simulink model "version13"  (Simulink 8.3)
settings: Solver=ode4  StartTime=0  StopTime=60  FixedStep=0.001  MaxStep=0.01  MinStep=0.005  RelTol=1e-3
values from neighbouring files (symbols this model uses):
  Actuator_Tg = 0.1    [init.m]
  airDensity = [1.225 1.0066 .81935 .66011 .52579 .41351 .31194 .22786 .16647 .12165 .08891 .040084 .01841 .0084634 .0039957 .0019663 .0010269 .0005681 .00030968 .00016321 .000082829 .000039921 .000018458 .0000082196 .000003416 .0000005604 .00000009708 .00000002222 .000000008152 .000000003831 .000000002076 .000000001233 .0000000007815 .0000000005194 .0000000003581 .0000000002541 .0000000001367 .00000000007858 .0 ...(+113 chars)    [init.m]
  alphaRange = [-30, -25, -20, -15, -12, -10, -8, -6, -4, -2, 0, 2, 4, 6, 8, 10, 12, 15, 20, 25, 30]    [init.m]
  betaRange = alphaRange    [init.m]
  Cmy_beta = Cmz_alpha    [init.m]
  Cz = Cy    [init.m]
  D = 0.122    [init.m]
  deltayRange = deltazRange    [init.m]
  deltazRange = [-20, -15, -10, -5, 0, 5, 10, 15, 20]    [init.m]
  fai0 = 0    [init.m]
  fai_v0 = 0    [init.m]
  g = 9.8    [init.m]
  gama0 = 0    [init.m]
  h = [0 2 4 6 8 10 12 14 16 18 20 25 30 35 40 45 50 55 60 65 70 75 80 85 90 100 110 120 130 140 150 160 170 180 190 200 220 240 260 280 300 400 500 600 700 800 900]    [init.m]
  Ixx = linspace(0.007,0.006,length(P))    [init.m]
  Iyy = linspace(1.0920,0.7440,length(P))    [init.m]
  K = 4    [init.m]
  Kd_ny = 5    [init.m]
  Kp_gamma = 5    [init.m]
  Kp_ny = 5    [init.m]
  Kp_nz = 5    [init.m]
  L = 1.2    [init.m]
  m = linspace(12+2,9.2,length(P))    [init.m]
  MachRange = [0.6, 1.2, 1.5, 1.8, 2.2]    [init.m]
  Mx_wx = zeros(1,11)    [init.m]
  My_wy = zeros(1,11)    [init.m]
  Mz_wz = zeros(1,11)    [init.m]
  P = 0:0.5:t_propshutdown    [init.m]
  sit0 = angle/57.3    (= 0.139616055846)    [init.m]
  Sref = 0.0038465    [init.m]
  t_change = 0:0.5:t_propshutdown    [init.m]
  t_masschange = 9.5    [init.m]
  t_propshutdown = 9.5    [init.m]
  Tg = 0.5    [init.m]
  theta0 = angle/57.3    (= 0.139616055846)    [init.m]
  V0 = 0.6*340    (= 204)    [init.m]
  Vt = 200    [init.m]
  wx0 = 0    [init.m]
  wy0 = 0    [init.m]
  wz0 = 0    [init.m]
  x0 = 0    [init.m]
  xt0 = 2500    [init.m]
  y0 = 5000    [init.m]
  yt0 = 5000    [init.m]
  z0 = 0    [init.m]
  zt0 = 0    [init.m]
undefined symbols (not defined in the file or in its folder): Cmz_alpha, Cx, Cy, earthRadius
settings Model: Creator=Administrator  LastModifiedBy=answer
settings SolverCC: InitialStep=0.005
settings OptimizationCC: ExpressionDepthLimit=2147483647  InitFltsAndDblsToZero=on
settings DebuggingCC: AlgebraicLoopMsg=none  SaveWithParameterizedLinksMsg=none  SignalResolutionControl=TryResolveAllWithWarning  MultiTaskDSMMsg=warning  MultiTaskCondExecSysMsg=none  FcnCallInpInsideContextMsg=UseLocalSettings
settings SFSimCC: SimParseCustomCode=off
settings RTWCC: IncludeERTFirstTime=on
settings GRTTargetCC: TargetFcnLib=ansi_tfl_tmw.mat

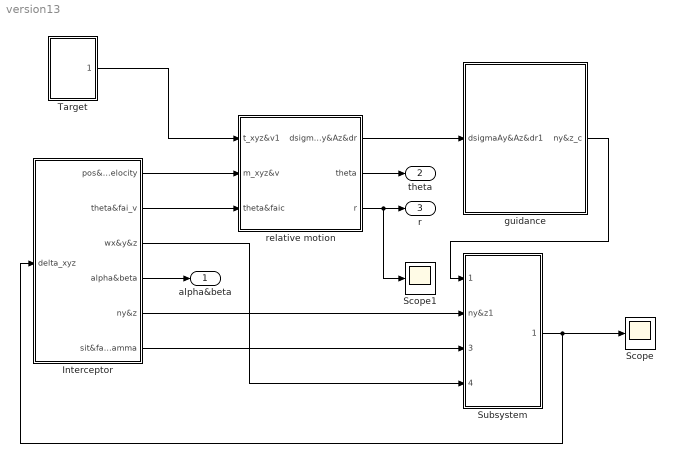
== system version13 ==
  Interceptor : Subsystem
  Scope : Scope
      settings: TimeRange=240  SaveName=ScopeData34
  Scope1 : Scope
      settings: TimeRange=240  SaveName=ScopeData41
  Subsystem : Subsystem
  Target : Subsystem
  guidance : Subsystem
  "relative motion " : Subsystem
  alpha&beta : Outport
  theta : Outport  Port=2
  r : Outport  Port=3
  wires:
  Subsystem/1("delta_xyz1 ") -> Interceptor/1(delta_xyz), Scope/1
  Interceptor/1(pos&velocity) -> "relative motion "/2(m_xyz&v)
  Interceptor/2(theta&fai_v) -> "relative motion "/3(theta&faic)
  Interceptor/4(alpha&beta) -> alpha&beta/1
  Target/1(t_xyz&v) -> "relative motion "/1(t_xyz&v1)
  "relative motion "/2(theta) -> theta/1
  "relative motion "/3(r) -> Scope1/1, r/1
  "relative motion "/1(dsigmaAy&Az&dr) -> guidance/1(dsigmaAy&Az&dr1)
  guidance/1(ny&z_c) -> Subsystem/1(ny&z_c1)
  Interceptor/5(ny&z) -> Subsystem/2("ny&z1 ")
  Interceptor/3(wx&y&z) -> Subsystem/4("wx&y&z1 ")
  Interceptor/6(sit&fai&gamma) -> Subsystem/3(sit&fai&gamma1)

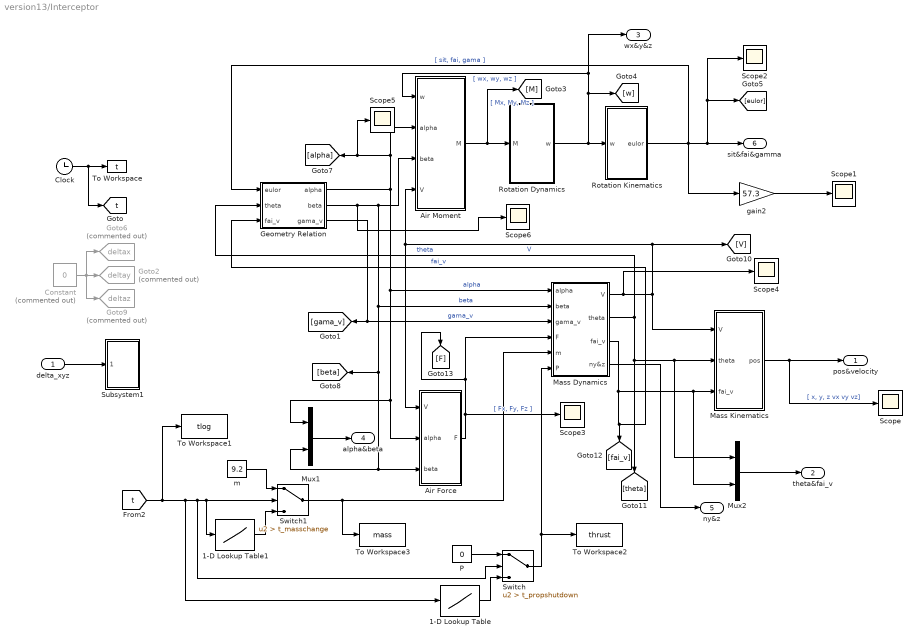
== system version13/Interceptor ==
  delta_xyz : Inport
  1-D Lookup Table : Lookup_n-D  NumberOfTableDimensions=1  BreakpointsForDimension1=t_change  Table=P  InternalRulePriority=Speed  RndMeth=Simplest  InputSameDT=on
  1-D Lookup Table1 : Lookup_n-D  NumberOfTableDimensions=1  BreakpointsForDimension1=t_change  Table=m  InternalRulePriority=Speed  RndMeth=Simplest  InputSameDT=on
  Air Force : Subsystem
  Air Moment : Subsystem
  Clock : Clock
  Constant : Constant  Commented=on  Value=0
  Geometry Relation : Subsystem
  Goto2 : Goto  Commented=on  GotoTag=deltay  TagVisibility=global
  Goto6 : Goto  Commented=on  GotoTag=deltax  TagVisibility=global
  Goto9 : Goto  Commented=on  GotoTag=deltaz  TagVisibility=global
  Mass Dynamics : Subsystem
  Mass Kinematics : Subsystem
  Mux1 : Mux  Inputs=2
  Mux2 : Mux  Inputs=2
  P : Constant  Value=0
  Rotation Dynamics : Subsystem
  Rotation Kinematics : Subsystem
  Scope{,1..6} (7 alike) : Scope
      Scope settings: TimeRange=240  SaveName=ScopeData6
      Scope1 settings: TimeRange=80  YMin=-50  YMax=30  SaveName=ScopeData13
      Scope2 settings: SaveName=ScopeData14
      Scope3 settings: SaveName=ScopeData15
      Scope4 settings: TimeRange=240  SaveName=ScopeData24
      Scope5 settings: TimeRange=80  YMin=-50  YMax=30  SaveName=ScopeData25
      Scope6 settings: TimeRange=60  YMin=-2  YMax=2  SaveName=ScopeData26
  Subsystem1 : Subsystem
  Switch : Switch  Criteria=u2 > Threshold  Threshold=t_propshutdown
  Switch1 : Switch  Criteria=u2 > Threshold  Threshold=t_masschange
  To Workspace : ToWorkspace  VariableName=t  SampleTime=-1
  To Workspace1 : ToWorkspace  VariableName=tlog  SampleTime=-1
  To Workspace2 : ToWorkspace  VariableName=thrust  SampleTime=-1
  To Workspace3 : ToWorkspace  VariableName=mass  SaveFormat=Timeseries  SampleTime=-1
  gain2 : Gain  Gain=57.3
  m : Constant  Value=9.2
  pos&velocity : Outport
  theta&fai_v : Outport  Port=2
  wx&y&z : Outport  Port=3
  alpha&beta : Outport  Port=4
  ny&z : Outport  Port=5
  sit&fai&gamma : Outport  Port=6
  tag scope: t=global
  wires:
  Mux1/1 -> alpha&beta/1
  delta_xyz/1 -> Subsystem1/1(delta_xyz)
  Constant/1 -> Goto6/1, Goto9/1, Goto2/1
  Mass Dynamics/4("ny&z ") -> ny&z/1
  Mass Dynamics/2(theta) -> [theta], Mux2/1, Mass Kinematics/2(theta), Geometry Relation/2(theta)  "theta"
  Air Moment/1(M) -> Rotation Dynamics/1(M), [M]  "[ Mx, My, Mz ]"
  Geometry Relation/3(gama_v) -> [gama_v], Mass Dynamics/3(gama_v)  "gama_v"
  m/1 -> Switch1/1
  Mux2/1 -> theta&fai_v/1
  gain2/1 -> Scope1/1
  P/1 -> Switch/1
  Geometry Relation/2(beta) -> Scope6/1, Mux1/2, Air Force/3(beta), [beta], Mass Dynamics/2(beta), Air Moment/3(beta)  "beta"
  1-D Lookup Table/1 -> Switch/3
  1-D Lookup Table1/1 -> Switch1/3
  [t] -> To Workspace1/1, 1-D Lookup Table/1, Switch/2, 1-D Lookup Table1/1, Switch1/2
  Rotation Kinematics/1(eulor) -> sit&fai&gamma/1, Scope2/1, [eulor], gain2/1, Geometry Relation/1(eulor)  "[ sit, fai, gama ]"
  Switch/1 -> To Workspace2/1, Mass Dynamics/6(P)
  Mass Kinematics/1(pos) -> pos&velocity/1, Scope/1  "[ x, y, z vx vy vz]"
  Switch1/1 -> To Workspace3/1, Mass Dynamics/5(m)
  Geometry Relation/1(alpha) -> Air Force/2(alpha), Mux1/1, Mass Dynamics/1(alpha), Air Moment/2(alpha), Scope5/1, [alpha]  "alpha"
  Air Force/1(F) -> Scope3/1, Mass Dynamics/4(F), [F]  "[ Fx, Fy, Fz ]"
  Mass Dynamics/1(V) -> Mass Kinematics/1(V), Air Moment/4(V), Air Force/1(V), [V], Scope4/1  "V"
  Mass Dynamics/3(fai_v) -> Geometry Relation/3(fai_v), [fai_v], Mux2/2, Mass Kinematics/3(" fai_v")  "fai_v"
  Rotation Dynamics/1(w) -> Rotation Kinematics/1(w), wx&y&z/1, Air Moment/1(w), [w]  "[ wx, wy, wz ]"
  Clock/1 -> [t], To Workspace/1

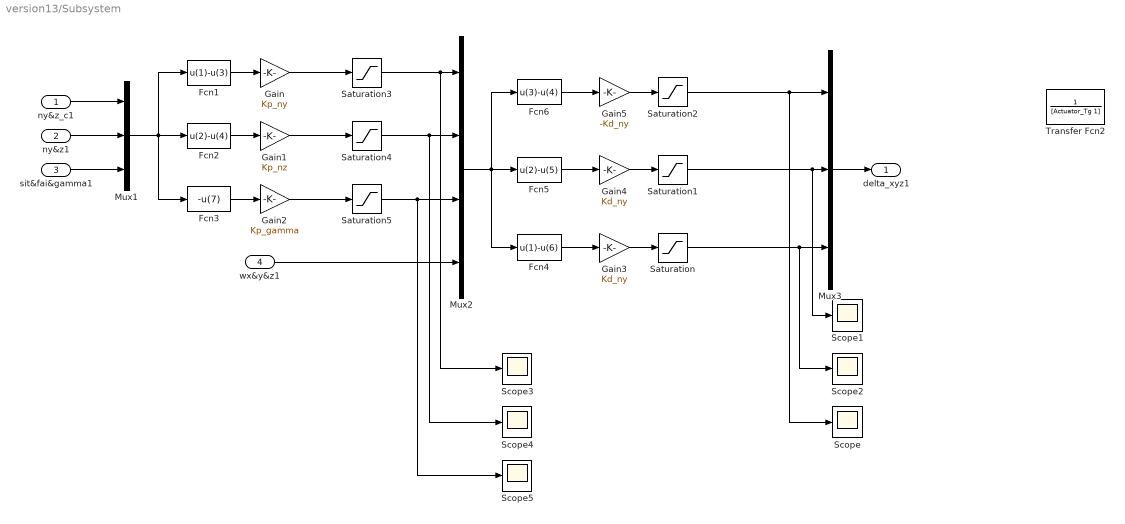
== system version13/Subsystem ==
  ny&z_c1 : Inport
  "ny&z1 " : Inport  Port=2
  sit&fai&gamma1 : Inport  Port=3
  "wx&y&z1 " : Inport  Port=4
  Fcn1 : Fcn  Expr=u(1)-u(3)
  Fcn2 : Fcn  Expr=u(2)-u(4)
  Fcn3 : Fcn  Expr=-u(7)
  Fcn4 : Fcn  Expr=u(1)-u(6)
  Fcn5 : Fcn  Expr=u(2)-u(5)
  Fcn6 : Fcn  Expr=u(3)-u(4)
  Gain : Gain  Gain=Kp_ny
  Gain1 : Gain  Gain=Kp_nz
  Gain2 : Gain  Gain=Kp_gamma
  Gain3 : Gain  Gain=Kd_ny
  Gain4 : Gain  Gain=Kd_ny
  Gain5 : Gain  Gain=-Kd_ny
  Mux1 : Mux  Inputs=3
  Mux2 : Mux
  Mux3 : Mux  Inputs=3
  Saturation{,1..5} (6 alike) : Saturate  UpperLimit=20  LowerLimit=-20
  Scope{,1..5} (6 alike) : Scope
      Scope settings: TimeRange=240  SaveName=ScopeData35
      Scope1 settings: TimeRange=240  SaveName=ScopeData36
      Scope2 settings: TimeRange=240  SaveName=ScopeData37
      Scope3 settings: TimeRange=240  SaveName=ScopeData38
      Scope4 settings: TimeRange=240  SaveName=ScopeData39
      Scope5 settings: TimeRange=240  SaveName=ScopeData40
  Transfer Fcn2 : TransferFcn  Denominator=[Actuator_Tg 1]
  "delta_xyz1 " : Outport
  wires:
  Fcn2/1 -> Gain1/1
  Fcn6/1 -> Gain5/1
  Fcn1/1 -> Gain/1
  Fcn5/1 -> Gain4/1
  Gain3/1 -> Saturation/1
  ny&z_c1/1 -> Mux1/1
  Fcn3/1 -> Gain2/1
  Gain4/1 -> Saturation1/1
  "ny&z1 "/1 -> Mux1/2
  Mux1/1 -> Fcn3/1, Fcn2/1, Fcn1/1
  sit&fai&gamma1/1 -> Mux1/3
  Gain5/1 -> Saturation2/1
  Fcn4/1 -> Gain3/1
  "wx&y&z1 "/1 -> Mux2/4
  Mux2/1 -> Fcn6/1, Fcn4/1, Fcn5/1
  Saturation1/1 -> Scope1/1, Mux3/2
  Mux3/1 -> "delta_xyz1 "/1
  Saturation/1 -> Scope2/1, Mux3/3
  Gain2/1 -> Saturation5/1
  Gain1/1 -> Saturation4/1
  Gain/1 -> Saturation3/1
  Saturation3/1 -> Scope3/1, Mux2/1
  Saturation4/1 -> Scope4/1, Mux2/2
  Saturation5/1 -> Scope5/1, Mux2/3
  Saturation2/1 -> Scope/1, Mux3/1

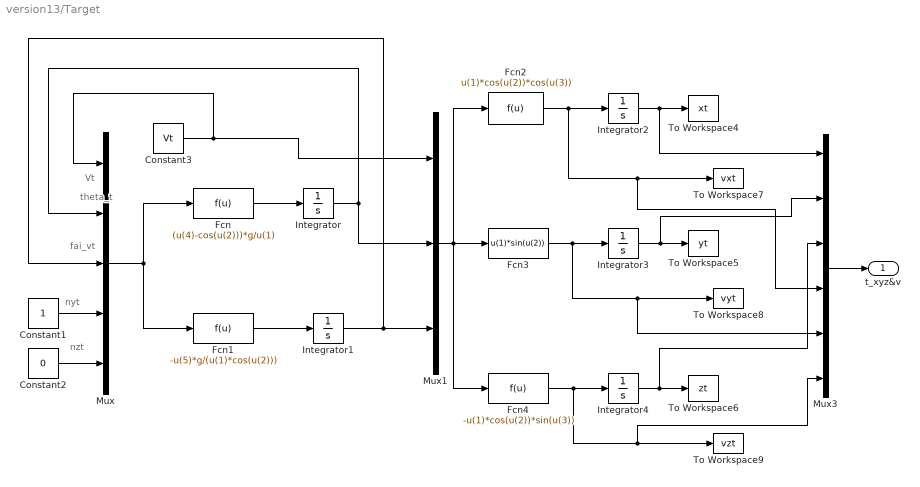
== system version13/Target ==
  note: nyt
  note: nzt
  note: Vt
  note: theta_t
  note: fai_vt
  Constant1 : Constant
  Constant2 : Constant  Value=0
  Constant3 : Constant  Value=Vt
  Fcn : Fcn  Expr=(u(4)-cos(u(2)))*g/u(1)
  Fcn1 : Fcn  Expr=-u(5)*g/(u(1)*cos(u(2)))
  Fcn2 : Fcn  Expr=u(1)*cos(u(2))*cos(u(3))
  Fcn3 : Fcn  Expr=u(1)*sin(u(2))
  Fcn4 : Fcn  Expr=-u(1)*cos(u(2))*sin(u(3))
  Integrator : Integrator
  Integrator1 : Integrator
  Integrator2 : Integrator  InitialCondition=xt0
  Integrator3 : Integrator  InitialCondition=yt0
  Integrator4 : Integrator  InitialCondition=zt0
  Mux : Mux  Inputs=5
  Mux1 : Mux  Inputs=3
  Mux3 : Mux  Inputs=6
  To Workspace4 : ToWorkspace  VariableName=xt  SampleTime=-1
  To Workspace5 : ToWorkspace  VariableName=yt  SampleTime=-1
  To Workspace6 : ToWorkspace  VariableName=zt  SampleTime=-1
  To Workspace7 : ToWorkspace  VariableName=vxt  SampleTime=-1
  To Workspace8 : ToWorkspace  VariableName=vyt  SampleTime=-1
  To Workspace9 : ToWorkspace  VariableName=vzt  SampleTime=-1
  t_xyz&v : Outport
  wires:
  Fcn2/1 -> Integrator2/1, Mux3/4, To Workspace7/1
  Mux/1 -> Fcn/1, Fcn1/1
  Constant2/1 -> Mux/5
  Mux1/1 -> Fcn2/1, Fcn3/1, Fcn4/1
  Fcn3/1 -> Mux3/5, To Workspace8/1, Integrator3/1
  Fcn4/1 -> Integrator4/1, Mux3/6, To Workspace9/1
  Integrator3/1 -> Mux3/2, To Workspace5/1
  Integrator2/1 -> Mux3/1, To Workspace4/1
  Integrator4/1 -> Mux3/3, To Workspace6/1
  Mux3/1 -> t_xyz&v/1
  Fcn1/1 -> Integrator1/1
  Constant3/1 -> Mux1/1, Mux/1
  Integrator1/1 -> Mux1/3, Mux/3
  Integrator/1 -> Mux1/2, Mux/2
  Fcn/1 -> Integrator/1
  Constant1/1 -> Mux/4

== system version13/guidance ==
  dsigmaAy&Az&dr1 : Inport
  Mux1 : Mux  Inputs=2
  Transfer Fcn : TransferFcn  Denominator=[Tg 1]
  Transfer Fcn1 : TransferFcn  Denominator=[Tg 1]
  ny : Fcn  Expr=K*u(2)*abs(u(3))/g
  nz : Fcn  Expr=-K*u(1)*abs(u[3])/g
  ny&z_c : Outport
  wires:
  dsigmaAy&Az&dr1/1 -> nz/1, ny/1
  nz/1 -> Transfer Fcn1/1
  Transfer Fcn1/1 -> Mux1/2
  ny/1 -> Transfer Fcn/1
  Mux1/1 -> ny&z_c/1
  Transfer Fcn/1 -> Mux1/1

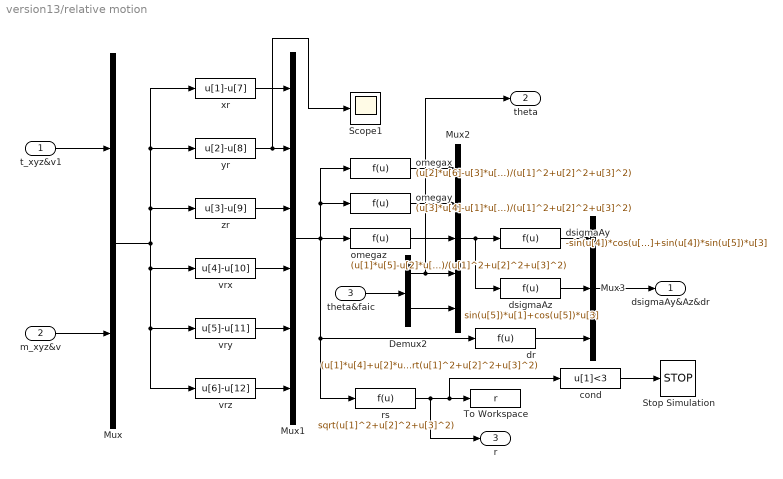
== system version13/relative motion  ==
  t_xyz&v1 : Inport
  m_xyz&v : Inport  Port=2
  theta&faic : Inport  Port=3
  Demux2 : Demux  Outputs=2
  Mux : Mux  Inputs=2
  Mux1 : Mux  Inputs=6
  Mux2 : Mux  Inputs=5
  Mux3 : Mux  Inputs=3
  Scope1 : Scope
      settings: TimeRange=240  SaveName=ScopeData42
  Stop Simulation : Stop
  To Workspace : ToWorkspace  VariableName=r  SampleTime=-1
  cond : Fcn  Expr=u[1]<3
  dr : Fcn  Expr=(u[1]*u[4]+u[2]*u[5]+u[3]*u[6])/sqrt(u[1]^2+u[2]^2+u[3]^2)
  dsigmaAy : Fcn  Expr=-sin(u[4])*cos(u[5])*u[1]+cos(u[4])*u[2]+sin(u[4])*sin(u[5])*u[3]
  dsigmaAz : Fcn  Expr=sin(u[5])*u[1]+cos(u[5])*u[3]
  omegax : Fcn  Expr=(u[2]*u[6]-u[3]*u[5])/(u[1]^2+u[2]^2+u[3]^2)
  omegay : Fcn  Expr=(u[3]*u[4]-u[1]*u[6])/(u[1]^2+u[2]^2+u[3]^2)
  omegaz : Fcn  Expr=(u[1]*u[5]-u[2]*u[4])/(u[1]^2+u[2]^2+u[3]^2)
  rs : Fcn  Expr=sqrt(u[1]^2+u[2]^2+u[3]^2)
  vrx : Fcn  Expr=u[4]-u[10]
  vry : Fcn  Expr=u[5]-u[11]
  vrz : Fcn  Expr=u[6]-u[12]
  xr : Fcn  Expr=u[1]-u[7]
  yr : Fcn  Expr=u[2]-u[8]
  zr : Fcn  Expr=u[3]-u[9]
  dsigmaAy&Az&dr : Outport
  theta : Outport  Port=2
  r : Outport  Port=3
  wires:
  yr/1 -> Scope1/1, Mux1/2
  xr/1 -> Mux1/1
  dsigmaAz/1 -> Mux3/2
  cond/1 -> Stop Simulation/1
  dsigmaAy/1 -> Mux3/1
  omegax/1 -> Mux2/1
  t_xyz&v1/1 -> Mux/1
  dr/1 -> Mux3/3
  vry/1 -> Mux1/5
  omegay/1 -> Mux2/2
  theta&faic/1 -> Demux2/1
  omegaz/1 -> Mux2/3
  Demux2/1 -> theta/1, Mux2/4
  Mux/1 -> xr/1, yr/1, zr/1, vrx/1, vrz/1, vry/1
  rs/1 -> r/1, cond/1, To Workspace/1
  vrx/1 -> Mux1/4
  m_xyz&v/1 -> Mux/2
  Mux1/1 -> omegaz/1, omegax/1, omegay/1, dr/1, rs/1
  Mux3/1 -> dsigmaAy&Az&dr/1
  zr/1 -> Mux1/3
  Demux2/2 -> Mux2/5
  Mux2/1 -> dsigmaAy/1, dsigmaAz/1
  vrz/1 -> Mux1/6

== system version13/Interceptor/Air Force ==
  V : Inport
  alpha : Inport  Port=2
  beta : Inport  Port=3
  Cruise Air Force : Subsystem
  F : Outport
  wires:
  V/1 -> Cruise Air Force/1(V)  "V"
  alpha/1 -> Cruise Air Force/2(alpha)  "alpha"
  beta/1 -> Cruise Air Force/3(beta)  "beta"
  Cruise Air Force/1(F) -> F/1

== system version13/Interceptor/Air Moment ==
  w : Inport
  alpha : Inport  Port=2
  beta : Inport  Port=3
  V : Inport  Port=4
  " Air Moment" : Subsystem
  Scope : Scope
      settings: SaveName=ScopeData2
  M : Outport
  wires:
  V/1 -> " Air Moment"/3(V)  "V"
  alpha/1 -> " Air Moment"/1(alpha)  "alpha"
  " Air Moment"/1(M) -> Scope/1, M/1
  w/1 -> " Air Moment"/4(w)  "w"
  beta/1 -> " Air Moment"/2(beta)  "beta"

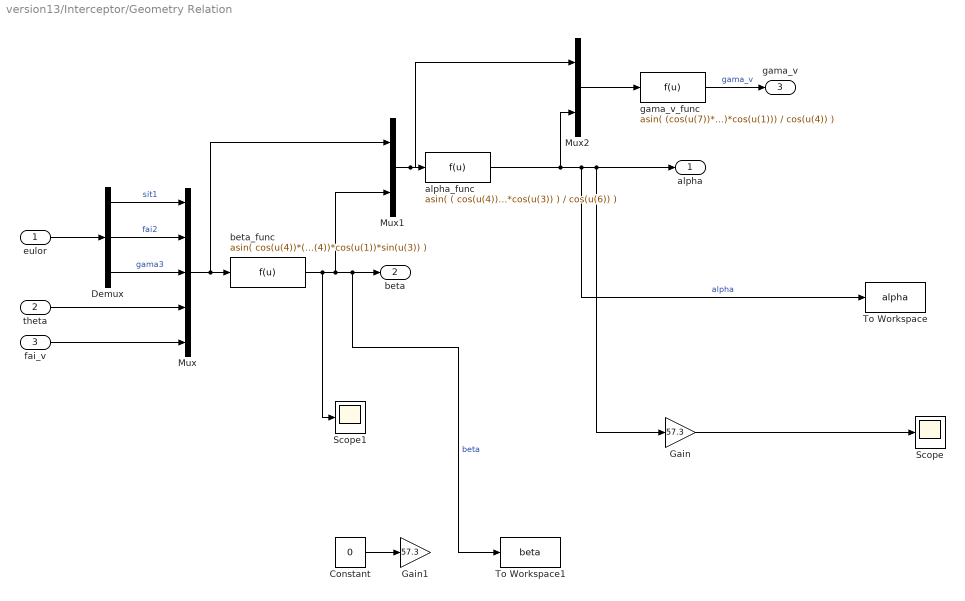
== system version13/Interceptor/Geometry Relation ==
  eulor : Inport
  theta : Inport  Port=2
  fai_v : Inport  Port=3
  Constant : Constant  Value=0
  Demux : Demux  Outputs=3
  Gain : Gain  Gain=57.3
  Gain1 : Gain  Gain=57.3
  Mux : Mux  Inputs=5
  Mux1 : Mux  Inputs=2
  Mux2 : Mux  Inputs=2
  Scope : Scope
  Scope1 : Scope
  To Workspace : ToWorkspace  VariableName=alpha  SampleTime=-1
  To Workspace1 : ToWorkspace  VariableName=beta  SampleTime=-1
  alpha_func : Fcn  Expr=asin( ( cos(u(4))*(sin(u(1))*cos(u(3))*cos(u(2)-u(5)) - sin(u(3))*sin(u(2)-u(5))) - sin(u(4))*cos(u(1))*cos(u(3)) ) / cos(u(6)) )
  beta_func : Fcn  Expr=asin( cos(u(4))*(cos(u(3))*sin(u(2)-u(5)) + sin(u(1))*sin(u(3))*cos(u(2)-u(5))) - sin(u(4))*cos(u(1))*sin(u(3)) )
  gama_v_func : Fcn  Expr=asin( (cos(u(7))*sin(u(6))*sin(u(1)) - sin(u(7))*sin(u(6))*cos(u(3))*cos(u(1)) + cos(u(6))*sin(u(3))*cos(u(1))) / cos(u(4)) )
  alpha : Outport
  beta : Outport  Port=2
  gama_v : Outport  Port=3
  wires:
  Demux/1 -> Mux/1  "sit1"
  Demux/2 -> Mux/2  "fai2"
  Demux/3 -> Mux/3  "gama3"
  eulor/1 -> Demux/1
  theta/1 -> Mux/4
  fai_v/1 -> Mux/5
  Mux/1 -> beta_func/1, Mux1/1
  beta_func/1 -> Scope1/1, To Workspace1/1, beta/1, Mux1/2  "beta"
  Mux1/1 -> Mux2/1, alpha_func/1
  alpha_func/1 -> To Workspace/1, Gain/1, alpha/1, Mux2/2  "alpha"
  Mux2/1 -> gama_v_func/1
  gama_v_func/1 -> gama_v/1  "gama_v"
  Gain/1 -> Scope/1
  Constant/1 -> Gain1/1

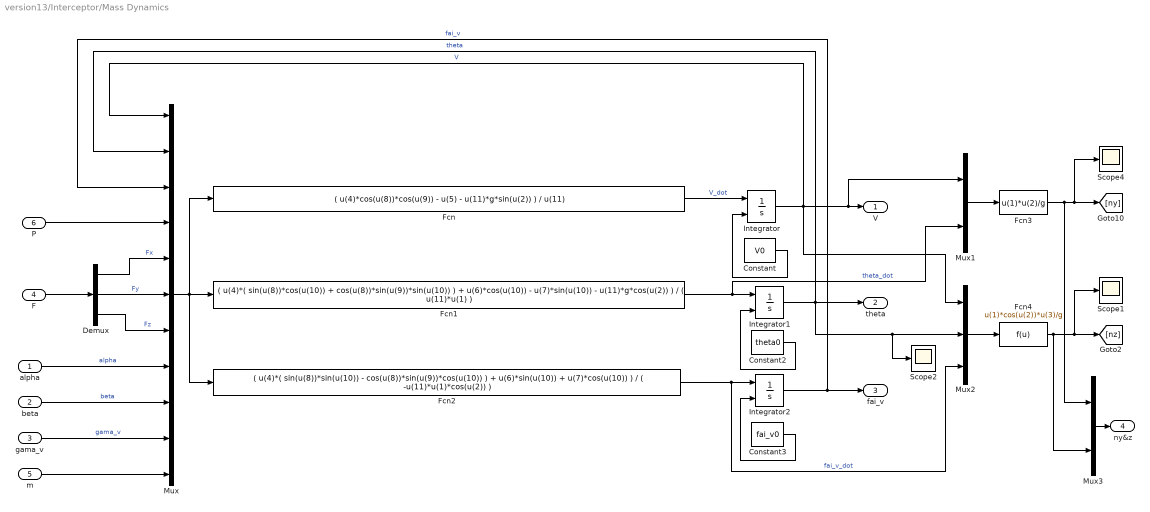
== system version13/Interceptor/Mass Dynamics ==
  alpha : Inport
  beta : Inport  Port=2
  gama_v : Inport  Port=3
  F : Inport  Port=4
  m : Inport  Port=5
  P : Inport  Port=6
  Constant : Constant  Value=V0
  Constant2 : Constant  Value=theta0
  Constant3 : Constant  Value=fai_v0
  Demux : Demux  Outputs=3
  Fcn : Fcn  Expr=( u(4)*cos(u(8))*cos(u(9)) - u(5) - u(11)*g*sin(u(2)) ) / u(11)
  Fcn1 : Fcn  Expr=( u(4)*( sin(u(8))*cos(u(10)) + cos(u(8))*sin(u(9))*sin(u(10)) ) + u(6)*cos(u(10)) - u(7)*sin(u(10)) - u(11)*g*cos(u(2)) ) / ( u(11)*u(1) )
  Fcn2 : Fcn  Expr=( u(4)*( sin(u(8))*sin(u(10)) - cos(u(8))*sin(u(9))*cos(u(10)) ) + u(6)*sin(u(10)) + u(7)*cos(u(10)) ) / ( -u(11)*u(1)*cos(u(2)) )
  Fcn3 : Fcn  Expr=u(1)*u(2)/g
  Fcn4 : Fcn  Expr=u(1)*cos(u(2))*u(3)/g
  Integrator : Integrator  InitialConditionSource=external
  Integrator1 : Integrator  InitialConditionSource=external
  Integrator2 : Integrator  InitialConditionSource=external
  Mux : Mux  Inputs=11
  Mux1 : Mux  Inputs=2
  Mux2 : Mux  Inputs=3
  Mux3 : Mux  Inputs=2
  Scope1 : Scope
      settings: TimeRange=240  SaveName=ScopeData32
  Scope2 : Scope
      settings: TimeRange=240  SaveName=ScopeData33
  Scope4 : Scope
      settings: TimeRange=240  SaveName=ScopeData31
  V : Outport
  theta : Outport  Port=2
  fai_v : Outport  Port=3
  "ny&z " : Outport  Port=4
  wires:
  Integrator/1 -> Mux2/1, Mux1/1, V/1, Mux/1  "V"
  Integrator1/1 -> Scope2/1, Mux2/2, theta/1, Mux/2  "theta"
  Integrator2/1 -> fai_v/1, Mux/3  "fai_v"
  Demux/2 -> Mux/6  "Fy"
  alpha/1 -> Mux/8  "alpha"
  beta/1 -> Mux/9  "beta"
  gama_v/1 -> Mux/10  "gama_v"
  Constant/1 -> Integrator/2
  Constant2/1 -> Integrator1/2
  Constant3/1 -> Integrator2/2
  Mux/1 -> Fcn1/1, Fcn/1, Fcn2/1
  Fcn2/1 -> Mux2/3, Integrator2/1  "fai_v_dot"
  Fcn/1 -> Integrator/1  "V_dot"
  Demux/1 -> Mux/5  "Fx"
  Demux/3 -> Mux/7  "Fz"
  F/1 -> Demux/1
  m/1 -> Mux/11
  P/1 -> Mux/4
  Fcn1/1 -> Mux1/2, Integrator1/1  "theta_dot"
  Mux1/1 -> Fcn3/1
  Fcn3/1 -> Mux3/1, Scope4/1, [ny]
  Mux2/1 -> Fcn4/1
  Fcn4/1 -> Mux3/2, Scope1/1, [nz]
  Mux3/1 -> "ny&z "/1

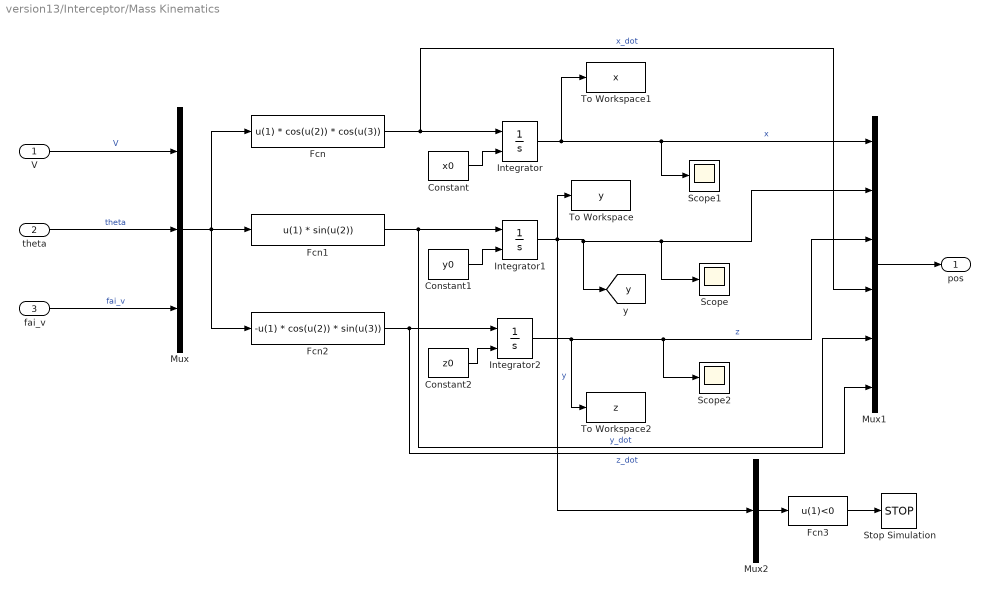
== system version13/Interceptor/Mass Kinematics ==
  V : Inport
  theta : Inport  Port=2
  " fai_v" : Inport  Port=3
  Constant : Constant  Value=x0
  Constant1 : Constant  Value=y0
  Constant2 : Constant  Value=z0
  Fcn : Fcn  Expr=u(1) * cos(u(2)) * cos(u(3))
  Fcn1 : Fcn  Expr=u(1) * sin(u(2))
  Fcn2 : Fcn  Expr=-u(1) * cos(u(2)) * sin(u(3))
  Fcn3 : Fcn  Expr=u(1)<0
  Integrator : Integrator  InitialConditionSource=external
  Integrator1 : Integrator  InitialConditionSource=external
  Integrator2 : Integrator  InitialConditionSource=external
  Mux : Mux  Inputs=3
  Mux1 : Mux  Inputs=6
  Mux2 : Mux  Inputs=1
  Scope : Scope
      settings: TimeRange=240  SaveName=ScopeData18
  Scope1 : Scope
      settings: TimeRange=240  SaveName=ScopeData19
  Scope2 : Scope
      settings: TimeRange=240  SaveName=ScopeData20
  Stop Simulation : Stop
  To Workspace : ToWorkspace  VariableName=y  SampleTime=-1
  To Workspace1 : ToWorkspace  VariableName=x  SampleTime=-1
  To Workspace2 : ToWorkspace  VariableName=z  SampleTime=-1
  pos : Outport
  tag scope: y=global
  wires:
  V/1 -> Mux/1  "V"
  theta/1 -> Mux/2  "theta"
  " fai_v"/1 -> Mux/3  "fai_v"
  Integrator1/1 -> Mux2/1, To Workspace/1, Scope/1, Mux1/2, [y]  "y"
  Constant/1 -> Integrator/2
  Constant1/1 -> Integrator1/2
  Constant2/1 -> Integrator2/2
  Fcn/1 -> Mux1/4, Integrator/1  "x_dot"
  Fcn1/1 -> Mux1/5, Integrator1/1  "y_dot"
  Fcn2/1 -> Mux1/6, Integrator2/1  "z_dot"
  Mux/1 -> Fcn1/1, Fcn/1, Fcn2/1
  Integrator2/1 -> Scope2/1, Mux1/3, To Workspace2/1  "z"
  Integrator/1 -> Scope1/1, Mux1/1, To Workspace1/1  "x"
  Mux2/1 -> Fcn3/1
  Fcn3/1 -> Stop Simulation/1
  Mux1/1 -> pos/1

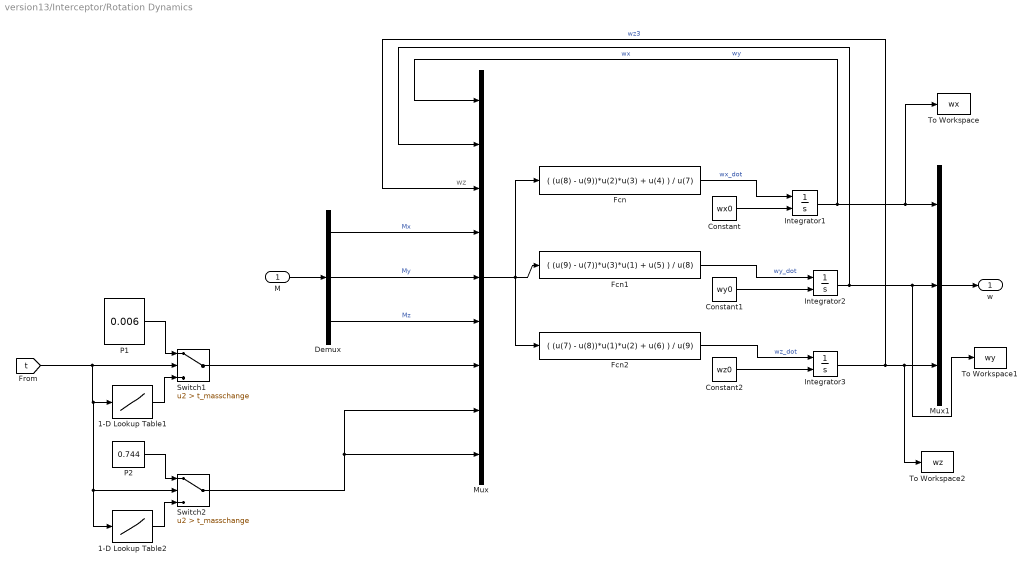
== system version13/Interceptor/Rotation Dynamics ==
  note: wz
  M : Inport
  1-D Lookup Table1 : Lookup_n-D  NumberOfTableDimensions=1  BreakpointsForDimension1=t_change  Table=Ixx  InternalRulePriority=Speed  RndMeth=Simplest  InputSameDT=on
  1-D Lookup Table2 : Lookup_n-D  NumberOfTableDimensions=1  BreakpointsForDimension1=t_change  Table=Iyy  InternalRulePriority=Speed  RndMeth=Simplest  InputSameDT=on
  Constant : Constant  Value=wx0
  Constant1 : Constant  Value=wy0
  Constant2 : Constant  Value=wz0
  Demux : Demux  Outputs=3
  Fcn : Fcn  Expr=( (u(8) - u(9))*u(2)*u(3) + u(4) ) / u(7)
  Fcn1 : Fcn  Expr=( (u(9) - u(7))*u(3)*u(1) + u(5) ) / u(8)
  Fcn2 : Fcn  Expr=( (u(7) - u(8))*u(1)*u(2) + u(6) ) / u(9)
  Integrator1 : Integrator  InitialConditionSource=external  InitialCondition=wy0
  Integrator2 : Integrator  InitialConditionSource=external  InitialCondition=wy0
  Integrator3 : Integrator  InitialConditionSource=external  InitialCondition=wz0
  Mux : Mux  Inputs=9
  Mux1 : Mux  Inputs=3
  P1 : Constant  Value=0.006
  P2 : Constant  Value=0.744
  Switch1 : Switch  Criteria=u2 > Threshold  Threshold=t_masschange
  Switch2 : Switch  Criteria=u2 > Threshold  Threshold=t_masschange
  To Workspace : ToWorkspace  VariableName=wx  SampleTime=-1
  To Workspace1 : ToWorkspace  VariableName=wy  SampleTime=-1
  To Workspace2 : ToWorkspace  VariableName=wz  SampleTime=-1
  w : Outport
  wires:
  Integrator1/1 -> Mux/1, To Workspace/1, Mux1/1  "wx"
  Integrator2/1 -> Mux/2, To Workspace1/1, Mux1/2  "wy"
  Integrator3/1 -> Mux/3, To Workspace2/1, Mux1/3  "wz3"
  Demux/3 -> Mux/6  "Mz"
  Demux/2 -> Mux/5  "My"
  Demux/1 -> Mux/4  "Mx"
  Mux/1 -> Fcn1/1, Fcn/1, Fcn2/1
  Constant/1 -> Integrator1/2
  Constant1/1 -> Integrator2/2
  Constant2/1 -> Integrator3/2
  M/1 -> Demux/1
  Mux1/1 -> w/1
  Fcn2/1 -> Integrator3/1  "wz_dot"
  Fcn1/1 -> Integrator2/1  "wy_dot"
  Fcn/1 -> Integrator1/1  "wx_dot"
  Switch2/1 -> Mux/9, Mux/8
  1-D Lookup Table1/1 -> Switch1/3
  P1/1 -> Switch1/1
  [t] -> Switch2/2, 1-D Lookup Table2/1, 1-D Lookup Table1/1, Switch1/2
  Switch1/1 -> Mux/7
  1-D Lookup Table2/1 -> Switch2/3
  P2/1 -> Switch2/1

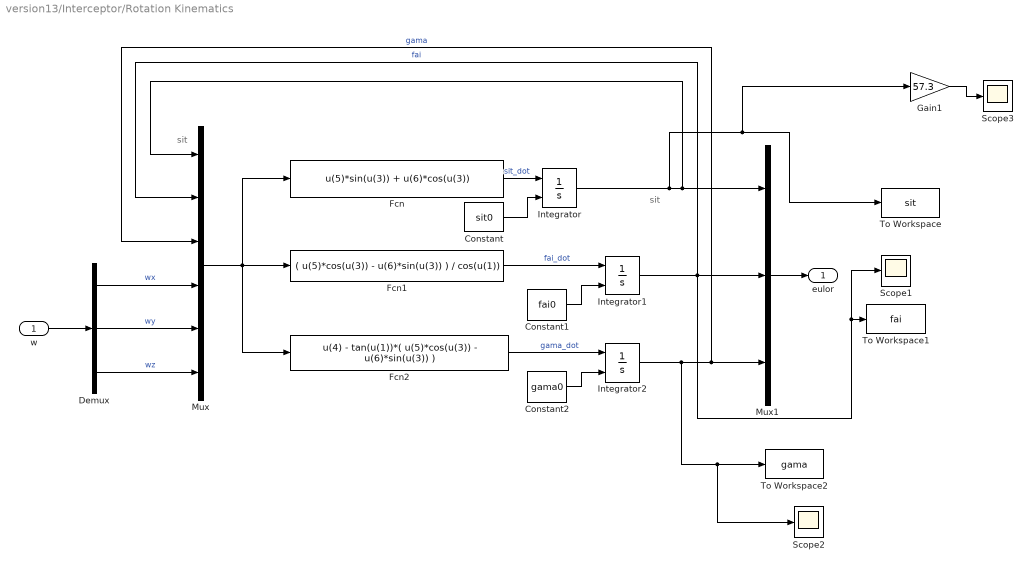
== system version13/Interceptor/Rotation Kinematics ==
  note: sit
  note: sit
  w : Inport
  Constant : Constant  Value=sit0
  Constant1 : Constant  Value=fai0
  Constant2 : Constant  Value=gama0
  Demux : Demux  Outputs=3
  Fcn : Fcn  Expr=u(5)*sin(u(3)) + u(6)*cos(u(3))
  Fcn1 : Fcn  Expr=( u(5)*cos(u(3)) - u(6)*sin(u(3)) ) / cos(u(1))
  Fcn2 : Fcn  Expr=u(4) - tan(u(1))*( u(5)*cos(u(3)) - u(6)*sin(u(3)) )
  Gain1 : Gain  Gain=57.3
  Integrator : Integrator  InitialConditionSource=external
  Integrator1 : Integrator  InitialConditionSource=external
  Integrator2 : Integrator  InitialConditionSource=external
  Mux : Mux  Inputs=6
  Mux1 : Mux  Inputs=3
  Scope1 : Scope
      settings: TimeRange=240  SaveName=ScopeData22
  Scope2 : Scope
      settings: TimeRange=240  SaveName=ScopeData23
  Scope3 : Scope
      settings: TimeRange=240  SaveName=ScopeData21
  To Workspace : ToWorkspace  VariableName=sit  SampleTime=-1
  To Workspace1 : ToWorkspace  VariableName=fai  SampleTime=-1
  To Workspace2 : ToWorkspace  VariableName=gama  SampleTime=-1
  eulor : Outport
  wires:
  Integrator1/1 -> Scope1/1, To Workspace1/1, Mux/2, Mux1/2  "fai"
  Integrator2/1 -> Scope2/1, To Workspace2/1, Mux/3, Mux1/3  "gama"
  Demux/1 -> Mux/4  "wx"
  Demux/2 -> Mux/5  "wy"
  Demux/3 -> Mux/6  "wz"
  Fcn/1 -> Integrator/1  "sit_dot"
  Fcn1/1 -> Integrator1/1  "fai_dot"
  Fcn2/1 -> Integrator2/1  "gama_dot"
  Constant2/1 -> Integrator2/2
  Constant1/1 -> Integrator1/2
  Constant/1 -> Integrator/2
  Mux/1 -> Fcn1/1, Fcn/1, Fcn2/1
  Mux1/1 -> eulor/1
  w/1 -> Demux/1
  Integrator/1 -> Gain1/1, To Workspace/1, Mux/1, Mux1/1
  Gain1/1 -> Scope3/1

== system version13/Interceptor/Subsystem1 ==
  delta_xyz : Inport
  Demux1 : Demux  Outputs=3
  tag scope: deltax=global, deltay=global, deltaz=global
  wires:
  Demux1/2 -> [deltay]
  Demux1/3 -> [deltaz]
  delta_xyz/1 -> Demux1/1
  Demux1/1 -> [deltax]

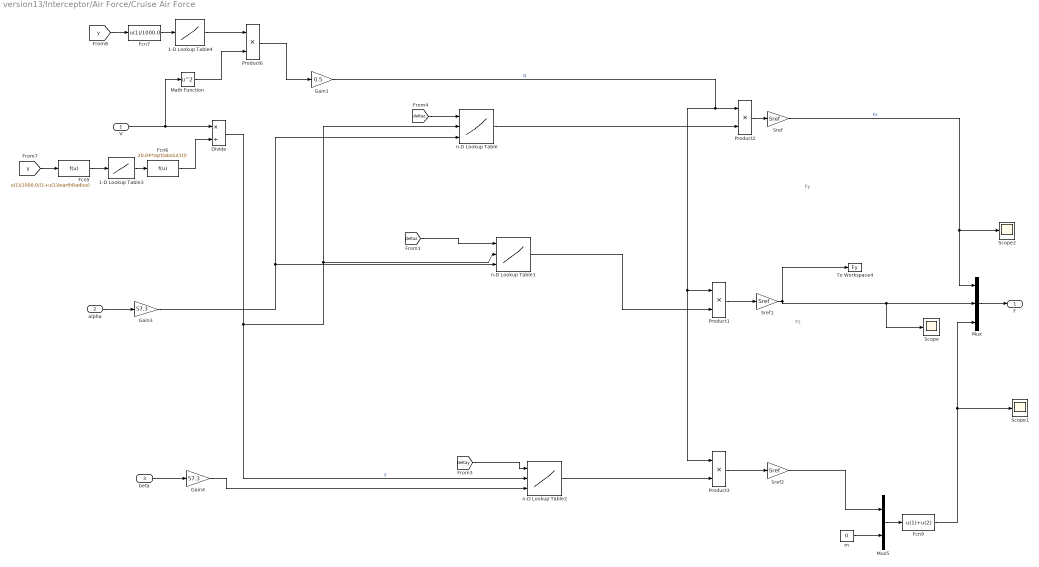
== system version13/Interceptor/Air Force/Cruise Air Force ==
  note: Fz
  note: Fy
  V : Inport
  alpha : Inport  Port=2
  beta : Inport  Port=3
  1-D Lookup Table3 : Lookup_n-D  NumberOfTableDimensions=1  BreakpointsForDimension1=[0 11.0 20.0 32.0 47.0 51.0 71.0 86.0]  Table=[288.15 216.65 216.65 228.65 270.65 270.65 214.65 186.95]  InternalRulePriority=Speed  RndMeth=Simplest  InputSameDT=on
  1-D Lookup Table4 : Lookup_n-D  NumberOfTableDimensions=1  BreakpointsForDimension1=h  Table=airDensity  InternalRulePriority=Speed  RndMeth=Simplest  InputSameDT=on
  Divide : Product  Inputs=*/
  Fcn5 : Fcn  Expr=u(1)/1000.0/(1+u(1)/earthRadius)
  Fcn6 : Fcn  Expr=20.04*sqrt(abs(u(1)))
  Fcn7 : Fcn  Expr=u(1)/1000.0
  Fcn9 : Fcn  Expr=u(1)+u(2)
  Gain1 : Gain  Gain=0.5
  Gain3 : Gain  Gain=57.3
  Gain4 : Gain  Gain=57.3
  Math Function : Math  Operator=square  SaturateOnIntegerOverflow=on
  Mux : Mux  Inputs=3
  Mux5 : Mux  Inputs=2
  Product{1..3,6} (4 alike) : Product  RndMeth=Zero
  Scope : Scope
      settings: SaveName=ScopeData10
  Scope1 : Scope
      settings: SaveName=ScopeData29
  Scope2 : Scope
      settings: SaveName=ScopeData30
  Sref : Gain  Gain=Sref
  Sref1 : Gain  Gain=Sref
  Sref2 : Gain  Gain=Sref
  To Workspace4 : ToWorkspace  VariableName=Fy  SampleTime=-1
  m : Constant  Value=0
  n-D Lookup Table : Lookup_n-D  NumberOfTableDimensions=3  BreakpointsForDimension1=deltazRange  BreakpointsForDimension2=MachRange  BreakpointsForDimension3=alphaRange  Table=Cx  InternalRulePriority=Speed  RndMeth=Simplest  InputSameDT=on
  n-D Lookup Table1 : Lookup_n-D  NumberOfTableDimensions=3  BreakpointsForDimension1=deltazRange  BreakpointsForDimension2=MachRange  BreakpointsForDimension3=alphaRange  Table=Cy  InternalRulePriority=Speed  RndMeth=Simplest  InputSameDT=on
  n-D Lookup Table2 : Lookup_n-D  NumberOfTableDimensions=3  BreakpointsForDimension1=deltayRange  BreakpointsForDimension2=MachRange  BreakpointsForDimension3=betaRange  Table=Cz  InternalRulePriority=Speed  RndMeth=Simplest  InputSameDT=on
  F : Outport
  wires:
  Product2/1 -> Sref/1
  V/1 -> Math Function/1, Divide/1
  Gain1/1 -> Product1/1, Product3/1, Product2/1  "Q"
  Math Function/1 -> Product6/2
  alpha/1 -> Gain3/1
  Mux/1 -> F/1
  Sref/1 -> Scope2/1, Mux/1  "Fx"
  beta/1 -> Gain4/1
  Sref2/1 -> Mux5/1
  Gain3/1 -> n-D Lookup Table/3, n-D Lookup Table1/3
  Sref1/1 -> Scope/1, Mux/2, To Workspace4/1
  n-D Lookup Table1/1 -> Product1/2
  n-D Lookup Table/1 -> Product2/2
  n-D Lookup Table2/1 -> Product3/2
  Product3/1 -> Sref2/1
  [y] -> Fcn7/1
  Fcn7/1 -> 1-D Lookup Table4/1
  1-D Lookup Table4/1 -> Product6/1
  Product6/1 -> Gain1/1
  [y] -> Fcn5/1
  Fcn5/1 -> 1-D Lookup Table3/1
  1-D Lookup Table3/1 -> Fcn6/1
  Fcn6/1 -> Divide/2
  Product1/1 -> Sref1/1
  Divide/1 -> n-D Lookup Table2/2, n-D Lookup Table1/2, n-D Lookup Table/2  "y"
  Mux5/1 -> Fcn9/1
  m/1 -> Mux5/2
  Fcn9/1 -> Scope1/1, Mux/3
  [deltaz] -> n-D Lookup Table1/1
  Gain4/1 -> n-D Lookup Table2/3
  [deltay] -> n-D Lookup Table2/1
  [deltaz] -> n-D Lookup Table/1

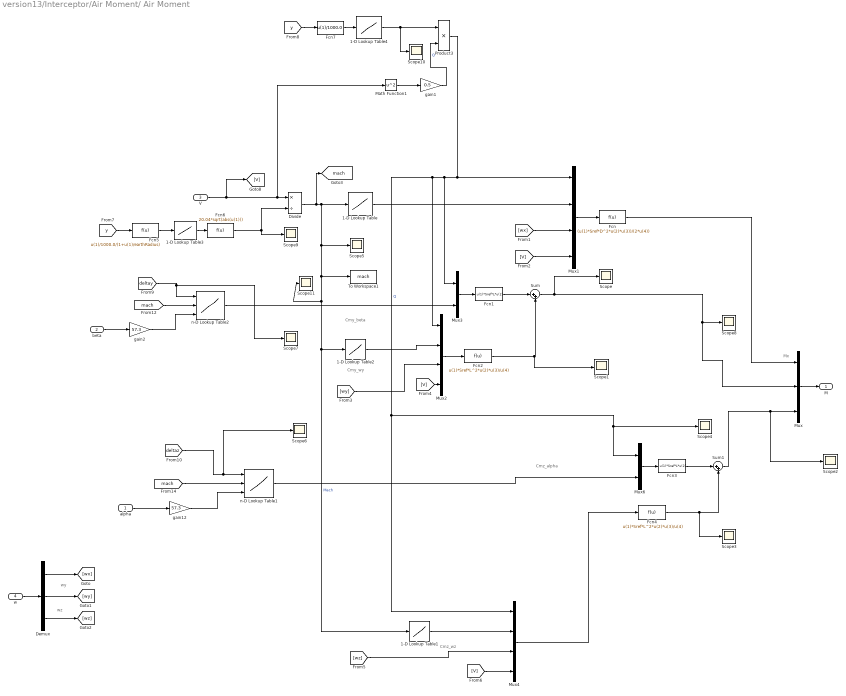
== system version13/Interceptor/Air Moment/ Air Moment ==
  note: Mx
  note: wz
  note: wy
  note: Cmy_wy
  note: Cmz_wz
  note: Cmy_beta
  note: Cmz_alpha
  alpha : Inport
  beta : Inport  Port=2
  V : Inport  Port=3
  w : Inport  Port=4
  1-D Lookup Table : Lookup_n-D  NumberOfTableDimensions=1  BreakpointsForDimension1=[0.4, 0.6, 0.8, 0.9, 1.0, 1.1, 1.2, 1.5, 2.0, 2.5, 3.0]  Table=Mx_wx  InternalRulePriority=Speed  RndMeth=Simplest  InputSameDT=on
  1-D Lookup Table1 : Lookup_n-D  NumberOfTableDimensions=1  BreakpointsForDimension1=[0.4 0.6 0.8 0.9 1 1.1 1.2 1.5 2 2.5 3]  Table=Mz_wz  InternalRulePriority=Speed  RndMeth=Simplest  InputSameDT=on
  1-D Lookup Table2 : Lookup_n-D  NumberOfTableDimensions=1  BreakpointsForDimension1=[0.4 0.6 0.8 0.9 1 1.1 1.2 1.5 2 2.5 3]  Table=My_wy  InternalRulePriority=Speed  RndMeth=Simplest  InputSameDT=on
  1-D Lookup Table3 : Lookup_n-D  NumberOfTableDimensions=1  BreakpointsForDimension1=[0 11.0 20.0 32.0 47.0 51.0 71.0 86.0]  Table=[288.15 216.65 216.65 228.65 270.65 270.65 214.65 186.95]  InternalRulePriority=Speed  RndMeth=Simplest  InputSameDT=on
  1-D Lookup Table4 : Lookup_n-D  NumberOfTableDimensions=1  BreakpointsForDimension1=h  Table=airDensity  InternalRulePriority=Speed  RndMeth=Simplest  InputSameDT=on
  Demux : Demux  Outputs=3
  Divide : Product  Inputs=*/
  Fcn : Fcn  Expr=(u(1)*Sref*D^2*u(2)*u(3))/(2*u(4))
  Fcn1 : Fcn  Expr=u(1)*Sref*L*u(2)
  Fcn2 : Fcn  Expr=u(1)*Sref*L^2*u(2)*u(3)/u(4)
  Fcn3 : Fcn  Expr=u(1)*Sref*L*u(2)
  Fcn4 : Fcn  Expr=u(1)*Sref*L^2*u(2)*u(3)/u(4)
  Fcn5 : Fcn  Expr=u(1)/1000.0/(1+u(1)/earthRadius)
  Fcn6 : Fcn  Expr=20.04*sqrt(abs(u(1)))
  Fcn7 : Fcn  Expr=u(1)/1000.0
  Math Function1 : Math  Operator=square  SaturateOnIntegerOverflow=on
  Mux : Mux  Inputs=3
  Mux1 : Mux
  Mux2 : Mux
  Mux3 : Mux  Inputs=2
  Mux4 : Mux
  Mux6 : Mux  Inputs=2
  Product3 : Product  RndMeth=Zero
  Scope{,1..11} (12 alike) : Scope
      Scope settings: SaveName=ScopeData3
      Scope1 settings: SaveName=ScopeData4
      Scope10 settings: SaveName=ScopeData17
      Scope11 settings: SaveName=ScopeData28
      Scope2 settings: SaveName=ScopeData5
      Scope3 settings: SaveName=ScopeData7
      Scope4 settings: SaveName=ScopeData8
      Scope5 settings: SaveName=ScopeData9
      Scope6 settings: SaveName=ScopeData11
      Scope7 settings: SaveName=ScopeData12
      Scope8 settings: YMin=-450  YMax=450  SaveName=ScopeData27
      Scope9 settings: SaveName=ScopeData16
  Sum : Sum  Inputs=|++
  Sum1 : Sum  Inputs=|++
  To Workspace1 : ToWorkspace  VariableName=mach  SampleTime=-1
  gain1 : Gain  Gain=0.5
  gain12 : Gain  Gain=57.3
  gain2 : Gain  Gain=57.3
  n-D Lookup Table1 : Lookup_n-D  NumberOfTableDimensions=3  BreakpointsForDimension1=deltazRange  BreakpointsForDimension2=MachRange  BreakpointsForDimension3=alphaRange  Table=Cmz_alpha  InternalRulePriority=Speed  RndMeth=Simplest  InputSameDT=on
  n-D Lookup Table2 : Lookup_n-D  NumberOfTableDimensions=3  BreakpointsForDimension1=deltayRange  BreakpointsForDimension2=MachRange  BreakpointsForDimension3=alphaRange  Table=Cmy_beta  InternalRulePriority=Speed  RndMeth=Simplest  InputSameDT=on
  M : Outport
  tag scope: mach=global
  wires:
  Mux/1 -> M/1
  Fcn6/1 -> Scope9/1, Divide/2
  Divide/1 -> [mach], 1-D Lookup Table/1, Scope5/1, Scope11/1, 1-D Lookup Table2/1, 1-D Lookup Table1/1, To Workspace1/1  "Mach"
  w/1 -> Demux/1
  Demux/1 -> [wx]
  Demux/2 -> [wy]
  Demux/3 -> [wz]
  Product3/1 -> Scope4/1, Mux6/1, Mux4/1, Mux2/1, Mux3/1, Mux1/1  "Q"
  1-D Lookup Table/1 -> Mux1/2
  [V] -> Mux1/4
  Mux1/1 -> Fcn/1
  [wx] -> Mux1/3
  Mux3/1 -> Fcn1/1
  [V] -> Mux2/4
  1-D Lookup Table2/1 -> Mux2/2
  Mux2/1 -> Fcn2/1
  Fcn1/1 -> Sum/1
  Fcn2/1 -> Scope1/1, Sum/2
  [V] -> Mux4/4
  Mux6/1 -> Fcn3/1
  Fcn3/1 -> Sum1/1
  Fcn4/1 -> Scope3/1, Sum1/2
  Mux4/1 -> Fcn4/1
  Sum1/1 -> Scope2/1, Mux/3
  Fcn/1 -> Mux/1
  1-D Lookup Table1/1 -> Mux4/2
  [wz] -> Mux4/3
  [wy] -> Mux2/3
  [y] -> Fcn5/1
  Fcn5/1 -> 1-D Lookup Table3/1
  1-D Lookup Table3/1 -> Fcn6/1
  V/1 -> Math Function1/1, Divide/1, [V]
  Math Function1/1 -> gain1/1
  gain1/1 -> Product3/2  "Q"
  [y] -> Fcn7/1
  Fcn7/1 -> 1-D Lookup Table4/1
  1-D Lookup Table4/1 -> Scope10/1, Product3/1
  n-D Lookup Table1/1 -> Mux6/2
  [mach] -> n-D Lookup Table1/2
  alpha/1 -> gain12/1
  beta/1 -> gain2/1
  Sum/1 -> Mux/2, Scope8/1, Scope/1
  [mach] -> n-D Lookup Table2/2
  gain2/1 -> n-D Lookup Table2/3
  gain12/1 -> n-D Lookup Table1/3
  [deltaz] -> Scope6/1, n-D Lookup Table1/1
  n-D Lookup Table2/1 -> Mux3/2
  [deltay] -> Scope7/1, n-D Lookup Table2/1
